simulink model "MK_Snowman"  (R2023b)
settings: Solver=FixedStepAuto  StartTime=0.0  StopTime=1  FixedStep=0.01  RelTol=1e-3
libraries: MK_Snowman_Lib x3, simulink x1
settings Model: Creator=mluser  LastModifiedBy=mluser

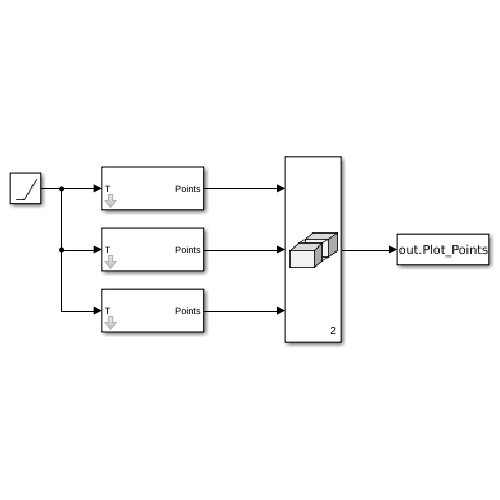
[thumbnail: Simulink's stored preview of the top-level diagram]
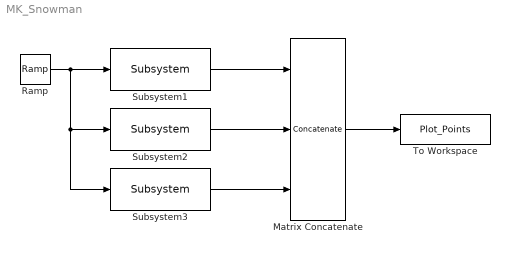
== system MK_Snowman ==
  Matrix Concatenate : Concatenate  NumInputs=3  Mode=Multidimensional array  ConcatenateDimension=2
  Ramp : simulink/Sources/Ramp  slope=1  start=0  InitialOutput=0
  Subsystem1 : MK_Snowman_Lib/Subsystem  A=1  B=1  X_Offset=0  Y_Offset=11
  Subsystem2 : MK_Snowman_Lib/Subsystem  A=2  B=2  X_Offset=0  Y_Offset=8
  Subsystem3 : MK_Snowman_Lib/Subsystem  A=3  B=3  X_Offset=0  Y_Offset=3
  To Workspace : ToWorkspace  VariableName=Plot_Points  SampleTime=-1
  wires:
  Ramp/1 -> Subsystem2/1, Subsystem3/1, Subsystem1/1
  Matrix Concatenate/1 -> To Workspace/1
  Subsystem1/1 -> Matrix Concatenate/1
  Subsystem2/1 -> Matrix Concatenate/2
  Subsystem3/1 -> Matrix Concatenate/3
